simulink model "Improved_version_succesful1"  (Simulink 7.3)
settings: Solver=ode45  StartTime=0.0  StopTime=.25  RelTol=1e-3
undefined symbols (not defined in the file or in its folder): x
libraries: powerlib x176, powerlib_extras x116
(part 2 of 3)

== system Improved_version_succesful1/compensation section3/compensation block ==
  vL : Inport  OutDataType=fixdt(1, 16)  OutScaling=2^0
  PL : Inport  Port=2  OutDataType=fixdt(1, 16)  OutScaling=2^0
  iL : Inport  Port=3  OutDataType=fixdt(1, 16)  OutScaling=2^0
  1 constant power : Subsystem
  1st- : powerlib_extras/Control  Blocks/1st-Order  Filter  DialogController=POWERSYS.PowerSysDialog  SystemSampleTime=-1  FilterType=Lowpass  Tc=.00051  Initialize=off  Vac_Init=[0.8 -25 60]  Vdc_Init=-0.4  PlotResponse=off  param1=[1 500 1]
  1st-O : powerlib_extras/Control  Blocks/1st-Order  Filter  DialogController=POWERSYS.PowerSysDialog  SystemSampleTime=-1  FilterType=Lowpass  Tc=.00051  Initialize=off  Vac_Init=[0.8 -25 60]  Vdc_Init=-0.4  PlotResponse=off  param1=[1 500 1]
  1st-Order  Filter{,1,3,5..6} (5 alike) : powerlib_extras/Control  Blocks/1st-Order  Filter  DialogController=POWERSYS.PowerSysDialog  SystemSampleTime=-1  FilterType=Lowpass  Tc=.00051  Initialize=off  Vac_Init=[0.8 -25 60]  Vdc_Init=-0.4  PlotResponse=off  param1=[1 500 1]
  2 unity PF : Subsystem
  "3 balanced currents " : Subsystem
  Demux1 : Demux  Outputs=3
  Demux2 : Demux  Outputs=3
  Gain : Gain  Gain=x(6)*(1-x(5))  ParameterDataType=fixdt(1, 16)  ParameterScaling=2^0  OutDataType=fixdt(1, 16)  OutScaling=2^0
  Gain1 : Gain  Gain=x(5)*(1-x(6))  ParameterDataType=fixdt(1, 16)  ParameterScaling=2^0  OutDataType=fixdt(1, 16)  OutScaling=2^0
  Gain2 : Gain  Gain=x(5)*x(6)  ParameterDataType=fixdt(1, 16)  ParameterScaling=2^0  OutDataType=fixdt(1, 16)  OutScaling=2^0
  Mux1 : Mux  Inputs=3
  Mux2 : Mux  Inputs=3
  Mux3 : Mux  Inputs=3
  Saturation1 : Saturate  UpperLimit=100  LowerLimit=-100  OutDataType=sfix(16)  OutScaling=2^0
  Saturation2 : Saturate  UpperLimit=10000  LowerLimit=0  OutDataType=sfix(16)  OutScaling=2^0
  Saturation3 : Saturate  UpperLimit=500  LowerLimit=-500  OutDataType=sfix(16)  OutScaling=2^0
  Scope : Scope  NumInputPorts=3
      settings: YMin=-7.5~-1~-1  YMax=10~1~1  SaveName=ScopeData33
  Sum : Sum  Inputs=|+++  OutDataType=fixdt(1, 16)  OutScaling=2^0
  Icomp. : Outport  OutDataType=sfix(16)  OutScaling=2^0
  wires:
  vL/1 -> Saturation3/1
  Demux1/1 -> 1st-/1
  Demux1/2 -> 1st-Order  Filter3/1
  Demux1/3 -> 1st-Order  Filter/1
  Saturation1/1 -> Demux1/1
  1st-Order  Filter1/1 -> Mux3/3
  Demux2/1 -> 1st-O/1
  Demux2/2 -> 1st-Order  Filter5/1
  Demux2/3 -> 1st-Order  Filter1/1
  1st-O/1 -> Mux3/1
  1st-Order  Filter5/1 -> Mux3/2
  Saturation2/1 -> 1st-Order  Filter6/1
  1st-/1 -> Mux2/1
  1st-Order  Filter3/1 -> Mux2/2
  1st-Order  Filter/1 -> Mux2/3
  Saturation3/1 -> Demux2/1
  iL/1 -> Saturation1/1
  PL/1 -> Saturation2/1
  Mux3/1 -> Mux1/2
  Mux2/1 -> Mux1/1
  1st-Order  Filter6/1 -> Mux1/3
  Gain/1 -> 1 constant power/1(In1)
  Mux1/1 -> Gain/1, Gain1/1, Gain2/1
  Gain1/1 -> 2 unity PF/1(In1)
  1 constant power/1(Out2) -> Sum/1, Scope/1
  2 unity PF/1(Out1) -> Sum/2, Scope/2
  Gain2/1 -> "3 balanced currents "/1(In1)
  "3 balanced currents "/1(iCabc) -> Sum/3, Scope/3
  Sum/1 -> Icomp./1

== system Improved_version_succesful1/compensation section4/compensation block ==
  vL : Inport  OutDataType=fixdt(1, 16)  OutScaling=2^0
  PL : Inport  Port=2  OutDataType=fixdt(1, 16)  OutScaling=2^0
  iL : Inport  Port=3  OutDataType=fixdt(1, 16)  OutScaling=2^0
  1 constant power : Subsystem
  1st- : powerlib_extras/Control  Blocks/1st-Order  Filter  DialogController=POWERSYS.PowerSysDialog  SystemSampleTime=-1  FilterType=Lowpass  Tc=.00051  Initialize=off  Vac_Init=[0.8 -25 60]  Vdc_Init=-0.4  PlotResponse=off  param1=[1 500 1]
  1st-O : powerlib_extras/Control  Blocks/1st-Order  Filter  DialogController=POWERSYS.PowerSysDialog  SystemSampleTime=-1  FilterType=Lowpass  Tc=.00051  Initialize=off  Vac_Init=[0.8 -25 60]  Vdc_Init=-0.4  PlotResponse=off  param1=[1 500 1]
  1st-Order  Filter{,1,3,5..6} (5 alike) : powerlib_extras/Control  Blocks/1st-Order  Filter  DialogController=POWERSYS.PowerSysDialog  SystemSampleTime=-1  FilterType=Lowpass  Tc=.00051  Initialize=off  Vac_Init=[0.8 -25 60]  Vdc_Init=-0.4  PlotResponse=off  param1=[1 500 1]
  2 unity PF : Subsystem
  "3 balanced currents " : Subsystem
  Demux1 : Demux  Outputs=3
  Demux2 : Demux  Outputs=3
  Gain : Gain  Gain=x(8)*(1-x(7))  ParameterDataType=fixdt(1, 16)  ParameterScaling=2^0  OutDataType=fixdt(1, 16)  OutScaling=2^0
  Gain1 : Gain  Gain=x(7)*(1-x(8))  ParameterDataType=fixdt(1, 16)  ParameterScaling=2^0  OutDataType=fixdt(1, 16)  OutScaling=2^0
  Gain2 : Gain  Gain=x(7)*x(8)  ParameterDataType=fixdt(1, 16)  ParameterScaling=2^0  OutDataType=fixdt(1, 16)  OutScaling=2^0
  Mux1 : Mux  Inputs=3
  Mux2 : Mux  Inputs=3
  Mux3 : Mux  Inputs=3
  Saturation1 : Saturate  UpperLimit=100  LowerLimit=-100  OutDataType=sfix(16)  OutScaling=2^0
  Saturation2 : Saturate  UpperLimit=10000  LowerLimit=0  OutDataType=sfix(16)  OutScaling=2^0
  Saturation3 : Saturate  UpperLimit=500  LowerLimit=-500  OutDataType=sfix(16)  OutScaling=2^0
  Scope : Scope  NumInputPorts=3
      settings: YMin=-7.5~-1~-1  YMax=10~1~1  SaveName=ScopeData33
  Sum : Sum  Inputs=|+++  OutDataType=fixdt(1, 16)  OutScaling=2^0
  Icomp. : Outport  OutDataType=sfix(16)  OutScaling=2^0
  wires:
  Sum/1 -> Icomp./1
  "3 balanced currents "/1(iCabc) -> Scope/3, Sum/3
  Gain2/1 -> "3 balanced currents "/1(In1)
  2 unity PF/1(Out1) -> Scope/2, Sum/2
  1 constant power/1(Out2) -> Scope/1, Sum/1
  Gain1/1 -> 2 unity PF/1(In1)
  Mux1/1 -> Gain2/1, Gain1/1, Gain/1
  Gain/1 -> 1 constant power/1(In1)
  1st-Order  Filter6/1 -> Mux1/3
  Mux2/1 -> Mux1/1
  Mux3/1 -> Mux1/2
  PL/1 -> Saturation2/1
  iL/1 -> Saturation1/1
  Saturation3/1 -> Demux2/1
  1st-Order  Filter/1 -> Mux2/3
  1st-Order  Filter3/1 -> Mux2/2
  1st-/1 -> Mux2/1
  Saturation2/1 -> 1st-Order  Filter6/1
  1st-Order  Filter5/1 -> Mux3/2
  1st-O/1 -> Mux3/1
  Demux2/3 -> 1st-Order  Filter1/1
  Demux2/2 -> 1st-Order  Filter5/1
  Demux2/1 -> 1st-O/1
  1st-Order  Filter1/1 -> Mux3/3
  Saturation1/1 -> Demux1/1
  Demux1/3 -> 1st-Order  Filter/1
  Demux1/2 -> 1st-Order  Filter3/1
  Demux1/1 -> 1st-/1
  vL/1 -> Saturation3/1

== system Improved_version_succesful1/compensation section5/compensation block ==
  vL : Inport  OutDataType=fixdt(1, 16)  OutScaling=2^0
  PL : Inport  Port=2  OutDataType=fixdt(1, 16)  OutScaling=2^0
  iL : Inport  Port=3  OutDataType=fixdt(1, 16)  OutScaling=2^0
  1 constant power : Subsystem
  1st- : powerlib_extras/Control  Blocks/1st-Order  Filter  DialogController=POWERSYS.PowerSysDialog  SystemSampleTime=-1  FilterType=Lowpass  Tc=.00051  Initialize=off  Vac_Init=[0.8 -25 60]  Vdc_Init=-0.4  PlotResponse=off  param1=[1 500 1]
  1st-O : powerlib_extras/Control  Blocks/1st-Order  Filter  DialogController=POWERSYS.PowerSysDialog  SystemSampleTime=-1  FilterType=Lowpass  Tc=.00051  Initialize=off  Vac_Init=[0.8 -25 60]  Vdc_Init=-0.4  PlotResponse=off  param1=[1 500 1]
  1st-Order  Filter{,1,3,5..6} (5 alike) : powerlib_extras/Control  Blocks/1st-Order  Filter  DialogController=POWERSYS.PowerSysDialog  SystemSampleTime=-1  FilterType=Lowpass  Tc=.00051  Initialize=off  Vac_Init=[0.8 -25 60]  Vdc_Init=-0.4  PlotResponse=off  param1=[1 500 1]
  2 unity PF : Subsystem
  "3 balanced currents " : Subsystem
  Demux1 : Demux  Outputs=3
  Demux2 : Demux  Outputs=3
  Gain : Gain  Gain=x(10)*(1-x(9))  ParameterDataType=fixdt(1, 16)  ParameterScaling=2^0  OutDataType=fixdt(1, 16)  OutScaling=2^0
  Gain1 : Gain  Gain=x(9)*(1-x(10))  ParameterDataType=fixdt(1, 16)  ParameterScaling=2^0  OutDataType=fixdt(1, 16)  OutScaling=2^0
  Gain2 : Gain  Gain=x(9)*x(10)  ParameterDataType=fixdt(1, 16)  ParameterScaling=2^0  OutDataType=fixdt(1, 16)  OutScaling=2^0
  Mux1 : Mux  Inputs=3
  Mux2 : Mux  Inputs=3
  Mux3 : Mux  Inputs=3
  Saturation1 : Saturate  UpperLimit=100  LowerLimit=-100  OutDataType=sfix(16)  OutScaling=2^0
  Saturation2 : Saturate  UpperLimit=10000  LowerLimit=0  OutDataType=sfix(16)  OutScaling=2^0
  Saturation3 : Saturate  UpperLimit=500  LowerLimit=-500  OutDataType=sfix(16)  OutScaling=2^0
  Scope : Scope  NumInputPorts=3
      settings: YMin=-7.5~-1~-1  YMax=10~1~1  SaveName=ScopeData33
  Sum : Sum  Inputs=|+++  OutDataType=fixdt(1, 16)  OutScaling=2^0
  Icomp. : Outport  OutDataType=sfix(16)  OutScaling=2^0
  wires:
  vL/1 -> Saturation3/1
  Demux1/1 -> 1st-/1
  Demux1/2 -> 1st-Order  Filter3/1
  Demux1/3 -> 1st-Order  Filter/1
  Saturation1/1 -> Demux1/1
  1st-Order  Filter1/1 -> Mux3/3
  Demux2/1 -> 1st-O/1
  Demux2/2 -> 1st-Order  Filter5/1
  Demux2/3 -> 1st-Order  Filter1/1
  1st-O/1 -> Mux3/1
  1st-Order  Filter5/1 -> Mux3/2
  Saturation2/1 -> 1st-Order  Filter6/1
  1st-/1 -> Mux2/1
  1st-Order  Filter3/1 -> Mux2/2
  1st-Order  Filter/1 -> Mux2/3
  Saturation3/1 -> Demux2/1
  iL/1 -> Saturation1/1
  PL/1 -> Saturation2/1
  Mux3/1 -> Mux1/2
  Mux2/1 -> Mux1/1
  1st-Order  Filter6/1 -> Mux1/3
  Gain/1 -> 1 constant power/1(In1)
  Mux1/1 -> Gain/1, Gain1/1, Gain2/1
  Gain1/1 -> 2 unity PF/1(In1)
  1 constant power/1(Out2) -> Sum/1, Scope/1
  2 unity PF/1(Out1) -> Sum/2, Scope/2
  Gain2/1 -> "3 balanced currents "/1(In1)
  "3 balanced currents "/1(iCabc) -> Sum/3, Scope/3
  Sum/1 -> Icomp./1

== system Improved_version_succesful1/compensation section1/compensation block/1 constant power ==
  In1 : Inport  OutDataType=fixdt(1, 16)  OutScaling=2^0
  Demux : Demux  Outputs=3
  Demux1 : Demux  Outputs=7
  Discrete  Mean value : powerlib_extras/Discrete Measurements/Discrete  Mean value  DialogController=POWERSYS.PowerSysDialog  SystemSampleTime=-1  Freq=50  Vinit=.001  Ts=50e-6
  Embedded MATLAB Function : Stateflow chart  TreatAsAtomicUnit=on
  Embedded MATLAB Function1 : Stateflow chart  TreatAsAtomicUnit=on
  Embedded MATLAB Function3 : Stateflow chart  TreatAsAtomicUnit=on
  Embedded MATLAB Function4 : Stateflow chart  TreatAsAtomicUnit=on
  Mux1 : Mux  Inputs=3
  Mux3 : Mux  Inputs=3
  Mux4 : Mux  Inputs=3
  Scope1 : Scope  NumInputPorts=3
      settings: YMin=-1~-1~-1  YMax=1~1~1  SaveName=ScopeData32
  Out2 : Outport  OutDataType=sfix(16)  OutScaling=2^0
  wires:
  Mux3/1 -> Embedded MATLAB Function/1(a)
  Mux4/1 -> Embedded MATLAB Function1/1(b)
  Embedded MATLAB Function3/1(y) -> Demux/1, Out2/1
  Embedded MATLAB Function4/1(y) -> Embedded MATLAB Function3/1(h)
  Mux1/1 -> Embedded MATLAB Function4/1(a)
  Discrete  Mean value/1 -> Mux1/2
  Embedded MATLAB Function1/1(y) -> Mux1/1
  Demux/3 -> Scope1/3
  Demux/2 -> Scope1/2
  Demux/1 -> Scope1/1
  Embedded MATLAB Function/1(y) -> Mux1/3
  In1/1 -> Demux1/1
  Demux1/1 -> Mux3/1
  Demux1/2 -> Mux3/2
  Demux1/3 -> Mux3/3
  Demux1/4 -> Mux4/1
  Demux1/5 -> Mux4/2
  Demux1/6 -> Mux4/3
  Demux1/7 -> Discrete  Mean value/1

== system Improved_version_succesful1/compensation section1/compensation block/2 unity PF ==
  In1 : Inport  OutDataType=fixdt(1, 16)  OutScaling=2^0
  Demux : Demux  Outputs=3
  Demux1 : Demux  Outputs=7
  Discrete  Mean value : powerlib_extras/Discrete Measurements/Discrete  Mean value  DialogController=POWERSYS.PowerSysDialog  SystemSampleTime=-1  Freq=50  Vinit=0  Ts=50e-6
  Discrete  Mean value1 : powerlib_extras/Discrete Measurements/Discrete  Mean value  DialogController=POWERSYS.PowerSysDialog  SystemSampleTime=-1  Freq=50  Vinit=0  Ts=50e-6
  Embedded MATLAB Function : Stateflow chart  TreatAsAtomicUnit=on
  Embedded MATLAB Function1 : Stateflow chart  TreatAsAtomicUnit=on
  Embedded MATLAB Function2 : Stateflow chart  TreatAsAtomicUnit=on
  Embedded MATLAB Function3 : Stateflow chart  TreatAsAtomicUnit=on
  Embedded MATLAB Function4 : Stateflow chart  TreatAsAtomicUnit=on
  Mux1 : Mux
  Mux3 : Mux  Inputs=3
  Mux4 : Mux  Inputs=3
  Scope : Scope  NumInputPorts=3
      settings: YMin=-1~-1~-1  YMax=1~1~1  SaveName=ScopeData31
  Out1 : Outport  OutDataType=sfix(16)  OutScaling=2^0
  wires:
  Embedded MATLAB Function1/1(y) -> Embedded MATLAB Function2/1(a), Mux1/2
  Demux1/7 -> Discrete  Mean value/1
  Mux4/1 -> Embedded MATLAB Function1/1(b)
  Mux3/1 -> Embedded MATLAB Function/1(a)
  Demux1/6 -> Mux4/3
  Demux1/5 -> Mux4/2
  Demux1/4 -> Mux4/1
  Demux1/3 -> Mux3/3
  Demux1/2 -> Mux3/2
  Demux1/1 -> Mux3/1
  In1/1 -> Demux1/1
  Embedded MATLAB Function/1(y) -> Mux1/1
  Discrete  Mean value1/1 -> Mux1/3
  Embedded MATLAB Function2/1(y) -> Discrete  Mean value1/1
  Embedded MATLAB Function3/1(y) -> Out1/1, Demux/1
  Embedded MATLAB Function4/1(y) -> Embedded MATLAB Function3/1(h)
  Mux1/1 -> Embedded MATLAB Function4/1(a)
  Discrete  Mean value/1 -> Mux1/4
  Demux/3 -> Scope/3
  Demux/2 -> Scope/2
  Demux/1 -> Scope/1

== system Improved_version_succesful1/compensation section1/compensation block/3 balanced currents  ==
  In1 : Inport  OutDataType=fixdt(1, 16)  OutScaling=2^0
  Demux1 : Demux  Outputs=7
  Embedded MATLAB Function : Stateflow chart  TreatAsAtomicUnit=on
  Embedded MATLAB Function2 : Stateflow chart  TreatAsAtomicUnit=on
  Embedded MATLAB Function3 : Stateflow chart  TreatAsAtomicUnit=on
  Mean Value : powerlib_extras/Measurements/Mean Value  DialogController=POWERSYS.PowerSysDialog  SystemSampleTime=-1  Period=1/60
  Mux2 : Mux
  Mux3 : Mux  Inputs=3
  Mux4 : Mux  Inputs=3
  Saturation : Saturate  UpperLimit=100  LowerLimit=-100  OutDataType=sfix(16)  OutScaling=2^0
  Scope : Scope  NumInputPorts=2
      settings: YMin=-200~-1  YMax=200~1  SaveName=ScopeData34
  Scope1 : Scope  NumInputPorts=3
      settings: YMin=-30~-500~0  YMax=25~500~7000  SaveName=ScopeData35
  e0ab+1 : MATLABFcn  MATLABFcn=[1/sqrt(3) 1/sqrt(3) 1/sqrt(3); sqrt(2)/sqrt(3) -1/sqrt(6) -1/sqrt(6); 0 1/sqrt(2) -1/sqrt(2)]*u
  positive sequence1 : Subsystem
  iCabc : Outport  OutDataType=fixdt(1, 16)  OutScaling=2^0
  wires:
  In1/1 -> Demux1/1
  Demux1/1 -> Mux3/1
  Demux1/2 -> Mux3/2
  Demux1/3 -> Mux3/3
  Demux1/4 -> Mux4/1
  Demux1/5 -> Mux4/2
  Demux1/6 -> Mux4/3
  Embedded MATLAB Function/1(iL_0dq) -> Mux2/1
  e0ab+1/1 -> Mux2/2
  Mean Value/1 -> Mux2/4
  Mux2/1 -> Embedded MATLAB Function2/1(u)
  Embedded MATLAB Function2/1(iL_0dq) -> Embedded MATLAB Function3/1(u)
  Embedded MATLAB Function3/1(y) -> Saturation/1
  positive sequence1/2(E+^2) -> Mux2/3
  positive sequence1/1(eabc1+) -> e0ab+1/1
  Saturation/1 -> iCabc/1, Scope/1
  Mux3/1 -> Embedded MATLAB Function/1(u), Scope1/1
  Mux4/1 -> positive sequence1/1(In1), Scope1/2
  Demux1/7 -> Mean Value/1, Scope1/3

== system Improved_version_succesful1/compensation section2/compensation block/1 constant power ==
  In1 : Inport  OutDataType=fixdt(1, 16)  OutScaling=2^0
  Demux : Demux  Outputs=3
  Demux1 : Demux  Outputs=7
  Discrete  Mean value : powerlib_extras/Discrete Measurements/Discrete  Mean value  DialogController=POWERSYS.PowerSysDialog  SystemSampleTime=-1  Freq=50  Vinit=.001  Ts=50e-6
  Embedded MATLAB Function : Stateflow chart  TreatAsAtomicUnit=on
  Embedded MATLAB Function1 : Stateflow chart  TreatAsAtomicUnit=on
  Embedded MATLAB Function3 : Stateflow chart  TreatAsAtomicUnit=on
  Embedded MATLAB Function4 : Stateflow chart  TreatAsAtomicUnit=on
  Mux1 : Mux  Inputs=3
  Mux3 : Mux  Inputs=3
  Mux4 : Mux  Inputs=3
  Scope1 : Scope  NumInputPorts=3
      settings: YMin=-1~-1~-1  YMax=1~1~1  SaveName=ScopeData32
  Out2 : Outport  OutDataType=sfix(16)  OutScaling=2^0
  wires:
  Demux1/7 -> Discrete  Mean value/1
  Demux1/6 -> Mux4/3
  Demux1/5 -> Mux4/2
  Demux1/4 -> Mux4/1
  Demux1/3 -> Mux3/3
  Demux1/2 -> Mux3/2
  Demux1/1 -> Mux3/1
  In1/1 -> Demux1/1
  Embedded MATLAB Function/1(y) -> Mux1/3
  Demux/1 -> Scope1/1
  Demux/2 -> Scope1/2
  Demux/3 -> Scope1/3
  Embedded MATLAB Function1/1(y) -> Mux1/1
  Discrete  Mean value/1 -> Mux1/2
  Mux1/1 -> Embedded MATLAB Function4/1(a)
  Embedded MATLAB Function4/1(y) -> Embedded MATLAB Function3/1(h)
  Embedded MATLAB Function3/1(y) -> Out2/1, Demux/1
  Mux4/1 -> Embedded MATLAB Function1/1(b)
  Mux3/1 -> Embedded MATLAB Function/1(a)

== system Improved_version_succesful1/compensation section2/compensation block/2 unity PF ==
  In1 : Inport  OutDataType=fixdt(1, 16)  OutScaling=2^0
  Demux : Demux  Outputs=3
  Demux1 : Demux  Outputs=7
  Discrete  Mean value : powerlib_extras/Discrete Measurements/Discrete  Mean value  DialogController=POWERSYS.PowerSysDialog  SystemSampleTime=-1  Freq=50  Vinit=0  Ts=50e-6
  Discrete  Mean value1 : powerlib_extras/Discrete Measurements/Discrete  Mean value  DialogController=POWERSYS.PowerSysDialog  SystemSampleTime=-1  Freq=50  Vinit=0  Ts=50e-6
  Embedded MATLAB Function : Stateflow chart  TreatAsAtomicUnit=on
  Embedded MATLAB Function1 : Stateflow chart  TreatAsAtomicUnit=on
  Embedded MATLAB Function2 : Stateflow chart  TreatAsAtomicUnit=on
  Embedded MATLAB Function3 : Stateflow chart  TreatAsAtomicUnit=on
  Embedded MATLAB Function4 : Stateflow chart  TreatAsAtomicUnit=on
  Mux1 : Mux
  Mux3 : Mux  Inputs=3
  Mux4 : Mux  Inputs=3
  Scope : Scope  NumInputPorts=3
      settings: YMin=-1~-1~-1  YMax=1~1~1  SaveName=ScopeData31
  Out1 : Outport  OutDataType=sfix(16)  OutScaling=2^0
  wires:
  Demux/1 -> Scope/1
  Demux/2 -> Scope/2
  Demux/3 -> Scope/3
  Discrete  Mean value/1 -> Mux1/4
  Mux1/1 -> Embedded MATLAB Function4/1(a)
  Embedded MATLAB Function4/1(y) -> Embedded MATLAB Function3/1(h)
  Embedded MATLAB Function3/1(y) -> Demux/1, Out1/1
  Embedded MATLAB Function2/1(y) -> Discrete  Mean value1/1
  Discrete  Mean value1/1 -> Mux1/3
  Embedded MATLAB Function/1(y) -> Mux1/1
  In1/1 -> Demux1/1
  Demux1/1 -> Mux3/1
  Demux1/2 -> Mux3/2
  Demux1/3 -> Mux3/3
  Demux1/4 -> Mux4/1
  Demux1/5 -> Mux4/2
  Demux1/6 -> Mux4/3
  Mux3/1 -> Embedded MATLAB Function/1(a)
  Mux4/1 -> Embedded MATLAB Function1/1(b)
  Demux1/7 -> Discrete  Mean value/1
  Embedded MATLAB Function1/1(y) -> Mux1/2, Embedded MATLAB Function2/1(a)

== system Improved_version_succesful1/compensation section2/compensation block/3 balanced currents  ==
  In1 : Inport  OutDataType=fixdt(1, 16)  OutScaling=2^0
  Demux1 : Demux  Outputs=7
  Embedded MATLAB Function : Stateflow chart  TreatAsAtomicUnit=on
  Embedded MATLAB Function2 : Stateflow chart  TreatAsAtomicUnit=on
  Embedded MATLAB Function3 : Stateflow chart  TreatAsAtomicUnit=on
  Mean Value : powerlib_extras/Measurements/Mean Value  DialogController=POWERSYS.PowerSysDialog  SystemSampleTime=-1  Period=1/60
  Mux2 : Mux
  Mux3 : Mux  Inputs=3
  Mux4 : Mux  Inputs=3
  Saturation : Saturate  UpperLimit=100  LowerLimit=-100  OutDataType=sfix(16)  OutScaling=2^0
  Scope : Scope  NumInputPorts=2
      settings: YMin=-200~-1  YMax=200~1  SaveName=ScopeData34
  Scope1 : Scope  NumInputPorts=3
      settings: YMin=-30~-500~0  YMax=25~500~7000  SaveName=ScopeData35
  e0ab+1 : MATLABFcn  MATLABFcn=[1/sqrt(3) 1/sqrt(3) 1/sqrt(3); sqrt(2)/sqrt(3) -1/sqrt(6) -1/sqrt(6); 0 1/sqrt(2) -1/sqrt(2)]*u
  positive sequence1 : Subsystem
  iCabc : Outport  OutDataType=fixdt(1, 16)  OutScaling=2^0
  wires:
  Demux1/7 -> Scope1/3, Mean Value/1
  Mux4/1 -> Scope1/2, positive sequence1/1(In1)
  Mux3/1 -> Scope1/1, Embedded MATLAB Function/1(u)
  Saturation/1 -> Scope/1, iCabc/1
  positive sequence1/1(eabc1+) -> e0ab+1/1
  positive sequence1/2(E+^2) -> Mux2/3
  Embedded MATLAB Function3/1(y) -> Saturation/1
  Embedded MATLAB Function2/1(iL_0dq) -> Embedded MATLAB Function3/1(u)
  Mux2/1 -> Embedded MATLAB Function2/1(u)
  Mean Value/1 -> Mux2/4
  e0ab+1/1 -> Mux2/2
  Embedded MATLAB Function/1(iL_0dq) -> Mux2/1
  Demux1/6 -> Mux4/3
  Demux1/5 -> Mux4/2
  Demux1/4 -> Mux4/1
  Demux1/3 -> Mux3/3
  Demux1/2 -> Mux3/2
  Demux1/1 -> Mux3/1
  In1/1 -> Demux1/1

== system Improved_version_succesful1/compensation section3/compensation block/1 constant power ==
  In1 : Inport  OutDataType=fixdt(1, 16)  OutScaling=2^0
  Demux : Demux  Outputs=3
  Demux1 : Demux  Outputs=7
  Discrete  Mean value : powerlib_extras/Discrete Measurements/Discrete  Mean value  DialogController=POWERSYS.PowerSysDialog  SystemSampleTime=-1  Freq=50  Vinit=.001  Ts=50e-6
  Embedded MATLAB Function : Stateflow chart  TreatAsAtomicUnit=on
  Embedded MATLAB Function1 : Stateflow chart  TreatAsAtomicUnit=on
  Embedded MATLAB Function3 : Stateflow chart  TreatAsAtomicUnit=on
  Embedded MATLAB Function4 : Stateflow chart  TreatAsAtomicUnit=on
  Mux1 : Mux  Inputs=3
  Mux3 : Mux  Inputs=3
  Mux4 : Mux  Inputs=3
  Scope1 : Scope  NumInputPorts=3
      settings: YMin=-1~-1~-1  YMax=1~1~1  SaveName=ScopeData32
  Out2 : Outport  OutDataType=sfix(16)  OutScaling=2^0
  wires:
  Mux3/1 -> Embedded MATLAB Function/1(a)
  Mux4/1 -> Embedded MATLAB Function1/1(b)
  Embedded MATLAB Function3/1(y) -> Demux/1, Out2/1
  Embedded MATLAB Function4/1(y) -> Embedded MATLAB Function3/1(h)
  Mux1/1 -> Embedded MATLAB Function4/1(a)
  Discrete  Mean value/1 -> Mux1/2
  Embedded MATLAB Function1/1(y) -> Mux1/1
  Demux/3 -> Scope1/3
  Demux/2 -> Scope1/2
  Demux/1 -> Scope1/1
  Embedded MATLAB Function/1(y) -> Mux1/3
  In1/1 -> Demux1/1
  Demux1/1 -> Mux3/1
  Demux1/2 -> Mux3/2
  Demux1/3 -> Mux3/3
  Demux1/4 -> Mux4/1
  Demux1/5 -> Mux4/2
  Demux1/6 -> Mux4/3
  Demux1/7 -> Discrete  Mean value/1

== system Improved_version_succesful1/compensation section3/compensation block/2 unity PF ==
  In1 : Inport  OutDataType=fixdt(1, 16)  OutScaling=2^0
  Demux : Demux  Outputs=3
  Demux1 : Demux  Outputs=7
  Discrete  Mean value : powerlib_extras/Discrete Measurements/Discrete  Mean value  DialogController=POWERSYS.PowerSysDialog  SystemSampleTime=-1  Freq=50  Vinit=0  Ts=50e-6
  Discrete  Mean value1 : powerlib_extras/Discrete Measurements/Discrete  Mean value  DialogController=POWERSYS.PowerSysDialog  SystemSampleTime=-1  Freq=50  Vinit=0  Ts=50e-6
  Embedded MATLAB Function : Stateflow chart  TreatAsAtomicUnit=on
  Embedded MATLAB Function1 : Stateflow chart  TreatAsAtomicUnit=on
  Embedded MATLAB Function2 : Stateflow chart  TreatAsAtomicUnit=on
  Embedded MATLAB Function3 : Stateflow chart  TreatAsAtomicUnit=on
  Embedded MATLAB Function4 : Stateflow chart  TreatAsAtomicUnit=on
  Mux1 : Mux
  Mux3 : Mux  Inputs=3
  Mux4 : Mux  Inputs=3
  Scope : Scope  NumInputPorts=3
      settings: YMin=-1~-1~-1  YMax=1~1~1  SaveName=ScopeData31
  Out1 : Outport  OutDataType=sfix(16)  OutScaling=2^0
  wires:
  Embedded MATLAB Function1/1(y) -> Embedded MATLAB Function2/1(a), Mux1/2
  Demux1/7 -> Discrete  Mean value/1
  Mux4/1 -> Embedded MATLAB Function1/1(b)
  Mux3/1 -> Embedded MATLAB Function/1(a)
  Demux1/6 -> Mux4/3
  Demux1/5 -> Mux4/2
  Demux1/4 -> Mux4/1
  Demux1/3 -> Mux3/3
  Demux1/2 -> Mux3/2
  Demux1/1 -> Mux3/1
  In1/1 -> Demux1/1
  Embedded MATLAB Function/1(y) -> Mux1/1
  Discrete  Mean value1/1 -> Mux1/3
  Embedded MATLAB Function2/1(y) -> Discrete  Mean value1/1
  Embedded MATLAB Function3/1(y) -> Out1/1, Demux/1
  Embedded MATLAB Function4/1(y) -> Embedded MATLAB Function3/1(h)
  Mux1/1 -> Embedded MATLAB Function4/1(a)
  Discrete  Mean value/1 -> Mux1/4
  Demux/3 -> Scope/3
  Demux/2 -> Scope/2
  Demux/1 -> Scope/1

== system Improved_version_succesful1/compensation section3/compensation block/3 balanced currents  ==
  In1 : Inport  OutDataType=fixdt(1, 16)  OutScaling=2^0
  Demux1 : Demux  Outputs=7
  Embedded MATLAB Function : Stateflow chart  TreatAsAtomicUnit=on
  Embedded MATLAB Function2 : Stateflow chart  TreatAsAtomicUnit=on
  Embedded MATLAB Function3 : Stateflow chart  TreatAsAtomicUnit=on
  Mean Value : powerlib_extras/Measurements/Mean Value  DialogController=POWERSYS.PowerSysDialog  SystemSampleTime=-1  Period=1/60
  Mux2 : Mux
  Mux3 : Mux  Inputs=3
  Mux4 : Mux  Inputs=3
  Saturation : Saturate  UpperLimit=100  LowerLimit=-100  OutDataType=sfix(16)  OutScaling=2^0
  Scope : Scope  NumInputPorts=2
      settings: YMin=-200~-1  YMax=200~1  SaveName=ScopeData34
  Scope1 : Scope  NumInputPorts=3
      settings: YMin=-30~-500~0  YMax=25~500~7000  SaveName=ScopeData35
  e0ab+1 : MATLABFcn  MATLABFcn=[1/sqrt(3) 1/sqrt(3) 1/sqrt(3); sqrt(2)/sqrt(3) -1/sqrt(6) -1/sqrt(6); 0 1/sqrt(2) -1/sqrt(2)]*u
  positive sequence1 : Subsystem
  iCabc : Outport  OutDataType=fixdt(1, 16)  OutScaling=2^0
  wires:
  In1/1 -> Demux1/1
  Demux1/1 -> Mux3/1
  Demux1/2 -> Mux3/2
  Demux1/3 -> Mux3/3
  Demux1/4 -> Mux4/1
  Demux1/5 -> Mux4/2
  Demux1/6 -> Mux4/3
  Embedded MATLAB Function/1(iL_0dq) -> Mux2/1
  e0ab+1/1 -> Mux2/2
  Mean Value/1 -> Mux2/4
  Mux2/1 -> Embedded MATLAB Function2/1(u)
  Embedded MATLAB Function2/1(iL_0dq) -> Embedded MATLAB Function3/1(u)
  Embedded MATLAB Function3/1(y) -> Saturation/1
  positive sequence1/2(E+^2) -> Mux2/3
  positive sequence1/1(eabc1+) -> e0ab+1/1
  Saturation/1 -> iCabc/1, Scope/1
  Mux3/1 -> Embedded MATLAB Function/1(u), Scope1/1
  Mux4/1 -> positive sequence1/1(In1), Scope1/2
  Demux1/7 -> Mean Value/1, Scope1/3

== system Improved_version_succesful1/compensation section4/compensation block/1 constant power ==
  In1 : Inport  OutDataType=fixdt(1, 16)  OutScaling=2^0
  Demux : Demux  Outputs=3
  Demux1 : Demux  Outputs=7
  Discrete  Mean value : powerlib_extras/Discrete Measurements/Discrete  Mean value  DialogController=POWERSYS.PowerSysDialog  SystemSampleTime=-1  Freq=50  Vinit=.001  Ts=50e-6
  Embedded MATLAB Function : Stateflow chart  TreatAsAtomicUnit=on
  Embedded MATLAB Function1 : Stateflow chart  TreatAsAtomicUnit=on
  Embedded MATLAB Function3 : Stateflow chart  TreatAsAtomicUnit=on
  Embedded MATLAB Function4 : Stateflow chart  TreatAsAtomicUnit=on
  Mux1 : Mux  Inputs=3
  Mux3 : Mux  Inputs=3
  Mux4 : Mux  Inputs=3
  Scope1 : Scope  NumInputPorts=3
      settings: YMin=-1~-1~-1  YMax=1~1~1  SaveName=ScopeData32
  Out2 : Outport  OutDataType=sfix(16)  OutScaling=2^0
  wires:
  Demux1/7 -> Discrete  Mean value/1
  Demux1/6 -> Mux4/3
  Demux1/5 -> Mux4/2
  Demux1/4 -> Mux4/1
  Demux1/3 -> Mux3/3
  Demux1/2 -> Mux3/2
  Demux1/1 -> Mux3/1
  In1/1 -> Demux1/1
  Embedded MATLAB Function/1(y) -> Mux1/3
  Demux/1 -> Scope1/1
  Demux/2 -> Scope1/2
  Demux/3 -> Scope1/3
  Embedded MATLAB Function1/1(y) -> Mux1/1
  Discrete  Mean value/1 -> Mux1/2
  Mux1/1 -> Embedded MATLAB Function4/1(a)
  Embedded MATLAB Function4/1(y) -> Embedded MATLAB Function3/1(h)
  Embedded MATLAB Function3/1(y) -> Out2/1, Demux/1
  Mux4/1 -> Embedded MATLAB Function1/1(b)
  Mux3/1 -> Embedded MATLAB Function/1(a)

== system Improved_version_succesful1/compensation section4/compensation block/2 unity PF ==
  In1 : Inport  OutDataType=fixdt(1, 16)  OutScaling=2^0
  Demux : Demux  Outputs=3
  Demux1 : Demux  Outputs=7
  Discrete  Mean value : powerlib_extras/Discrete Measurements/Discrete  Mean value  DialogController=POWERSYS.PowerSysDialog  SystemSampleTime=-1  Freq=50  Vinit=0  Ts=50e-6
  Discrete  Mean value1 : powerlib_extras/Discrete Measurements/Discrete  Mean value  DialogController=POWERSYS.PowerSysDialog  SystemSampleTime=-1  Freq=50  Vinit=0  Ts=50e-6
  Embedded MATLAB Function : Stateflow chart  TreatAsAtomicUnit=on
  Embedded MATLAB Function1 : Stateflow chart  TreatAsAtomicUnit=on
  Embedded MATLAB Function2 : Stateflow chart  TreatAsAtomicUnit=on
  Embedded MATLAB Function3 : Stateflow chart  TreatAsAtomicUnit=on
  Embedded MATLAB Function4 : Stateflow chart  TreatAsAtomicUnit=on
  Mux1 : Mux
  Mux3 : Mux  Inputs=3
  Mux4 : Mux  Inputs=3
  Scope : Scope  NumInputPorts=3
      settings: YMin=-1~-1~-1  YMax=1~1~1  SaveName=ScopeData31
  Out1 : Outport  OutDataType=sfix(16)  OutScaling=2^0
  wires:
  Demux/1 -> Scope/1
  Demux/2 -> Scope/2
  Demux/3 -> Scope/3
  Discrete  Mean value/1 -> Mux1/4
  Mux1/1 -> Embedded MATLAB Function4/1(a)
  Embedded MATLAB Function4/1(y) -> Embedded MATLAB Function3/1(h)
  Embedded MATLAB Function3/1(y) -> Demux/1, Out1/1
  Embedded MATLAB Function2/1(y) -> Discrete  Mean value1/1
  Discrete  Mean value1/1 -> Mux1/3
  Embedded MATLAB Function/1(y) -> Mux1/1
  In1/1 -> Demux1/1
  Demux1/1 -> Mux3/1
  Demux1/2 -> Mux3/2
  Demux1/3 -> Mux3/3
  Demux1/4 -> Mux4/1
  Demux1/5 -> Mux4/2
  Demux1/6 -> Mux4/3
  Mux3/1 -> Embedded MATLAB Function/1(a)
  Mux4/1 -> Embedded MATLAB Function1/1(b)
  Demux1/7 -> Discrete  Mean value/1
  Embedded MATLAB Function1/1(y) -> Mux1/2, Embedded MATLAB Function2/1(a)

== system Improved_version_succesful1/compensation section4/compensation block/3 balanced currents  ==
  In1 : Inport  OutDataType=fixdt(1, 16)  OutScaling=2^0
  Demux1 : Demux  Outputs=7
  Embedded MATLAB Function : Stateflow chart  TreatAsAtomicUnit=on
  Embedded MATLAB Function2 : Stateflow chart  TreatAsAtomicUnit=on
  Embedded MATLAB Function3 : Stateflow chart  TreatAsAtomicUnit=on
  Mean Value : powerlib_extras/Measurements/Mean Value  DialogController=POWERSYS.PowerSysDialog  SystemSampleTime=-1  Period=1/60
  Mux2 : Mux
  Mux3 : Mux  Inputs=3
  Mux4 : Mux  Inputs=3
  Saturation : Saturate  UpperLimit=100  LowerLimit=-100  OutDataType=sfix(16)  OutScaling=2^0
  Scope : Scope  NumInputPorts=2
      settings: YMin=-200~-1  YMax=200~1  SaveName=ScopeData34
  Scope1 : Scope  NumInputPorts=3
      settings: YMin=-30~-500~0  YMax=25~500~7000  SaveName=ScopeData35
  e0ab+1 : MATLABFcn  MATLABFcn=[1/sqrt(3) 1/sqrt(3) 1/sqrt(3); sqrt(2)/sqrt(3) -1/sqrt(6) -1/sqrt(6); 0 1/sqrt(2) -1/sqrt(2)]*u
  positive sequence1 : Subsystem
  iCabc : Outport  OutDataType=fixdt(1, 16)  OutScaling=2^0
  wires:
  Demux1/7 -> Scope1/3, Mean Value/1
  Mux4/1 -> Scope1/2, positive sequence1/1(In1)
  Mux3/1 -> Scope1/1, Embedded MATLAB Function/1(u)
  Saturation/1 -> Scope/1, iCabc/1
  positive sequence1/1(eabc1+) -> e0ab+1/1
  positive sequence1/2(E+^2) -> Mux2/3
  Embedded MATLAB Function3/1(y) -> Saturation/1
  Embedded MATLAB Function2/1(iL_0dq) -> Embedded MATLAB Function3/1(u)
  Mux2/1 -> Embedded MATLAB Function2/1(u)
  Mean Value/1 -> Mux2/4
  e0ab+1/1 -> Mux2/2
  Embedded MATLAB Function/1(iL_0dq) -> Mux2/1
  Demux1/6 -> Mux4/3
  Demux1/5 -> Mux4/2
  Demux1/4 -> Mux4/1
  Demux1/3 -> Mux3/3
  Demux1/2 -> Mux3/2
  Demux1/1 -> Mux3/1
  In1/1 -> Demux1/1

== system Improved_version_succesful1/compensation section5/compensation block/1 constant power ==
  In1 : Inport  OutDataType=fixdt(1, 16)  OutScaling=2^0
  Demux : Demux  Outputs=3
  Demux1 : Demux  Outputs=7
  Discrete  Mean value : powerlib_extras/Discrete Measurements/Discrete  Mean value  DialogController=POWERSYS.PowerSysDialog  SystemSampleTime=-1  Freq=50  Vinit=.001  Ts=50e-6
  Embedded MATLAB Function : Stateflow chart  TreatAsAtomicUnit=on
  Embedded MATLAB Function1 : Stateflow chart  TreatAsAtomicUnit=on
  Embedded MATLAB Function3 : Stateflow chart  TreatAsAtomicUnit=on
  Embedded MATLAB Function4 : Stateflow chart  TreatAsAtomicUnit=on
  Mux1 : Mux  Inputs=3
  Mux3 : Mux  Inputs=3
  Mux4 : Mux  Inputs=3
  Scope1 : Scope  NumInputPorts=3
      settings: YMin=-1~-1~-1  YMax=1~1~1  SaveName=ScopeData32
  Out2 : Outport  OutDataType=sfix(16)  OutScaling=2^0
  wires:
  Mux3/1 -> Embedded MATLAB Function/1(a)
  Mux4/1 -> Embedded MATLAB Function1/1(b)
  Embedded MATLAB Function3/1(y) -> Demux/1, Out2/1
  Embedded MATLAB Function4/1(y) -> Embedded MATLAB Function3/1(h)
  Mux1/1 -> Embedded MATLAB Function4/1(a)
  Discrete  Mean value/1 -> Mux1/2
  Embedded MATLAB Function1/1(y) -> Mux1/1
  Demux/3 -> Scope1/3
  Demux/2 -> Scope1/2
  Demux/1 -> Scope1/1
  Embedded MATLAB Function/1(y) -> Mux1/3
  In1/1 -> Demux1/1
  Demux1/1 -> Mux3/1
  Demux1/2 -> Mux3/2
  Demux1/3 -> Mux3/3
  Demux1/4 -> Mux4/1
  Demux1/5 -> Mux4/2
  Demux1/6 -> Mux4/3
  Demux1/7 -> Discrete  Mean value/1

== system Improved_version_succesful1/compensation section5/compensation block/2 unity PF ==
  In1 : Inport  OutDataType=fixdt(1, 16)  OutScaling=2^0
  Demux : Demux  Outputs=3
  Demux1 : Demux  Outputs=7
  Discrete  Mean value : powerlib_extras/Discrete Measurements/Discrete  Mean value  DialogController=POWERSYS.PowerSysDialog  SystemSampleTime=-1  Freq=50  Vinit=0  Ts=50e-6
  Discrete  Mean value1 : powerlib_extras/Discrete Measurements/Discrete  Mean value  DialogController=POWERSYS.PowerSysDialog  SystemSampleTime=-1  Freq=50  Vinit=0  Ts=50e-6
  Embedded MATLAB Function : Stateflow chart  TreatAsAtomicUnit=on
  Embedded MATLAB Function1 : Stateflow chart  TreatAsAtomicUnit=on
  Embedded MATLAB Function2 : Stateflow chart  TreatAsAtomicUnit=on
  Embedded MATLAB Function3 : Stateflow chart  TreatAsAtomicUnit=on
  Embedded MATLAB Function4 : Stateflow chart  TreatAsAtomicUnit=on
  Mux1 : Mux
  Mux3 : Mux  Inputs=3
  Mux4 : Mux  Inputs=3
  Scope : Scope  NumInputPorts=3
      settings: YMin=-1~-1~-1  YMax=1~1~1  SaveName=ScopeData31
  Out1 : Outport  OutDataType=sfix(16)  OutScaling=2^0
  wires:
  Embedded MATLAB Function1/1(y) -> Embedded MATLAB Function2/1(a), Mux1/2
  Demux1/7 -> Discrete  Mean value/1
  Mux4/1 -> Embedded MATLAB Function1/1(b)
  Mux3/1 -> Embedded MATLAB Function/1(a)
  Demux1/6 -> Mux4/3
  Demux1/5 -> Mux4/2
  Demux1/4 -> Mux4/1
  Demux1/3 -> Mux3/3
  Demux1/2 -> Mux3/2
  Demux1/1 -> Mux3/1
  In1/1 -> Demux1/1
  Embedded MATLAB Function/1(y) -> Mux1/1
  Discrete  Mean value1/1 -> Mux1/3
  Embedded MATLAB Function2/1(y) -> Discrete  Mean value1/1
  Embedded MATLAB Function3/1(y) -> Out1/1, Demux/1
  Embedded MATLAB Function4/1(y) -> Embedded MATLAB Function3/1(h)
  Mux1/1 -> Embedded MATLAB Function4/1(a)
  Discrete  Mean value/1 -> Mux1/4
  Demux/3 -> Scope/3
  Demux/2 -> Scope/2
  Demux/1 -> Scope/1

== system Improved_version_succesful1/compensation section5/compensation block/3 balanced currents  ==
  In1 : Inport  OutDataType=fixdt(1, 16)  OutScaling=2^0
  Demux1 : Demux  Outputs=7
  Embedded MATLAB Function : Stateflow chart  TreatAsAtomicUnit=on
  Embedded MATLAB Function2 : Stateflow chart  TreatAsAtomicUnit=on
  Embedded MATLAB Function3 : Stateflow chart  TreatAsAtomicUnit=on
  Mean Value : powerlib_extras/Measurements/Mean Value  DialogController=POWERSYS.PowerSysDialog  SystemSampleTime=-1  Period=1/60
  Mux2 : Mux
  Mux3 : Mux  Inputs=3
  Mux4 : Mux  Inputs=3
  Saturation : Saturate  UpperLimit=100  LowerLimit=-100  OutDataType=sfix(16)  OutScaling=2^0
  Scope : Scope  NumInputPorts=2
      settings: YMin=-200~-1  YMax=200~1  SaveName=ScopeData34
  Scope1 : Scope  NumInputPorts=3
      settings: YMin=-30~-500~0  YMax=25~500~7000  SaveName=ScopeData35
  e0ab+1 : MATLABFcn  MATLABFcn=[1/sqrt(3) 1/sqrt(3) 1/sqrt(3); sqrt(2)/sqrt(3) -1/sqrt(6) -1/sqrt(6); 0 1/sqrt(2) -1/sqrt(2)]*u
  positive sequence1 : Subsystem
  iCabc : Outport  OutDataType=fixdt(1, 16)  OutScaling=2^0
  wires:
  In1/1 -> Demux1/1
  Demux1/1 -> Mux3/1
  Demux1/2 -> Mux3/2
  Demux1/3 -> Mux3/3
  Demux1/4 -> Mux4/1
  Demux1/5 -> Mux4/2
  Demux1/6 -> Mux4/3
  Embedded MATLAB Function/1(iL_0dq) -> Mux2/1
  e0ab+1/1 -> Mux2/2
  Mean Value/1 -> Mux2/4
  Mux2/1 -> Embedded MATLAB Function2/1(u)
  Embedded MATLAB Function2/1(iL_0dq) -> Embedded MATLAB Function3/1(u)
  Embedded MATLAB Function3/1(y) -> Saturation/1
  positive sequence1/2(E+^2) -> Mux2/3
  positive sequence1/1(eabc1+) -> e0ab+1/1
  Saturation/1 -> iCabc/1, Scope/1
  Mux3/1 -> Embedded MATLAB Function/1(u), Scope1/1
  Mux4/1 -> positive sequence1/1(In1), Scope1/2
  Demux1/7 -> Mean Value/1, Scope1/3

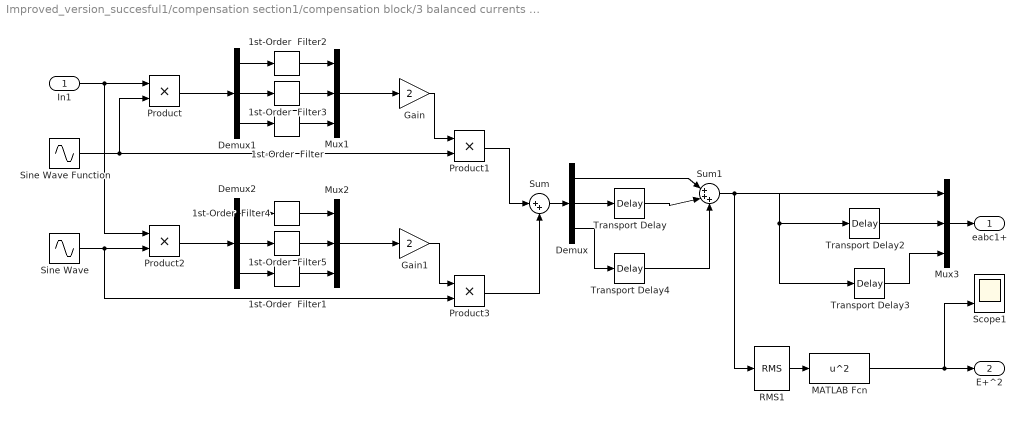
== system Improved_version_succesful1/compensation section1/compensation block/3 balanced currents /positive sequence1 ==
  In1 : Inport  OutDataType=sfix(16)  OutScaling=2^0
  1st-Order  Filter{,1,3,5} (4 alike) : powerlib_extras/Control  Blocks/1st-Order  Filter  DialogController=POWERSYS.PowerSysDialog  SystemSampleTime=-1  FilterType=Lowpass  Tc=.01  Initialize=off  Vac_Init=[0.8 -25 60]  Vdc_Init=-0.4  PlotResponse=off  param1=[1 500 1]
  1st-Order  Filter2 : powerlib_extras/Control  Blocks/1st-Order  Filter  DialogController=POWERSYS.PowerSysDialog  SystemSampleTime=-1  FilterType=Lowpass  Tc=.015  Initialize=off  Vac_Init=[0.8 -25 60]  Vdc_Init=-0.4  PlotResponse=off  param1=[1 500 1]
  1st-Order  Filter4 : powerlib_extras/Control  Blocks/1st-Order  Filter  DialogController=POWERSYS.PowerSysDialog  SystemSampleTime=-1  FilterType=Lowpass  Tc=.015  Initialize=off  Vac_Init=[0.8 -25 60]  Vdc_Init=-0.4  PlotResponse=off  param1=[1 500 1]
  Demux : Demux  Outputs=3
  Demux1 : Demux  Outputs=3
  Demux2 : Demux  Outputs=3
  Gain : Gain  Gain=2  ParameterDataType=sfix(16)  ParameterScaling=2^0  OutDataType=sfix(16)  OutScaling=2^0
  Gain1 : Gain  Gain=2  ParameterDataType=sfix(16)  ParameterScaling=2^0  OutDataType=sfix(16)  OutScaling=2^0
  MATLAB Fcn : MATLABFcn  MATLABFcn=u^2
  Mux1 : Mux  Inputs=3
  Mux2 : Mux  Inputs=3
  Mux3 : Mux  Inputs=3
  Product{,1..3} (4 alike) : Product  OutDataType=sfix(16)  OutScaling=2^0  RndMeth=Zero
  RMS1 : powerlib_extras/Measurements/RMS  DialogController=POWERSYS.PowerSysDialog  SystemSampleTime=-1  f1=50
  Scope1 : Scope  NumInputPorts=3
      settings: YMin=-1~-1~150000  YMax=1~1~320000
  Sine Wave : Sin  Amplitude=1  Bias=0  Frequency=100*pi  Phase=pi/2  Samples=10  SampleTime=0  Offset=0
  Sine Wave Function : Sin  Amplitude=1  Bias=0  Frequency=100*pi  Phase=0  Samples=10  SampleTime=0  Offset=0
  Sum : Sum  Inputs=|++  OutDataType=sfix(16)  OutScaling=2^0
  Sum1 : Sum  Inputs=|+++  OutDataType=sfix(16)  OutScaling=2^0
  Transport Delay : TransportDelay  DelayTime=.04/3
  Transport Delay2 : TransportDelay  DelayTime=.02/3
  Transport Delay3 : TransportDelay  DelayTime=.04/3
  Transport Delay4 : TransportDelay  DelayTime=.02/3
  eabc1+ : Outport  OutDataType=sfix(16)  OutScaling=2^0
  E+^2 : Outport  Port=2  OutDataType=sfix(16)  OutScaling=2^0
  wires:
  RMS1/1 -> MATLAB Fcn/1
  MATLAB Fcn/1 -> E+^2/1, Scope1/3
  In1/1 -> Product/1, Product2/1
  Sine Wave Function/1 -> Product/2, Product1/2
  1st-Order  Filter/1 -> Mux1/3
  Gain/1 -> Product1/1
  Sine Wave/1 -> Product2/2, Product3/2
  Gain1/1 -> Product3/1
  Product1/1 -> Sum/1
  Product3/1 -> Sum/2
  Sum/1 -> Demux/1
  Demux/2 -> Transport Delay/1
  Sum1/1 -> Transport Delay3/1, Mux3/1, RMS1/1, Transport Delay2/1
  Demux/3 -> Transport Delay4/1
  Transport Delay2/1 -> Mux3/2
  Transport Delay3/1 -> Mux3/3
  Mux3/1 -> eabc1+/1
  Demux1/1 -> 1st-Order  Filter2/1
  Demux1/2 -> 1st-Order  Filter3/1
  Demux1/3 -> 1st-Order  Filter/1
  Product/1 -> Demux1/1
  1st-Order  Filter2/1 -> Mux1/1
  1st-Order  Filter3/1 -> Mux1/2
  Mux1/1 -> Gain/1
  1st-Order  Filter1/1 -> Mux2/3
  Demux2/1 -> 1st-Order  Filter4/1
  Demux2/2 -> 1st-Order  Filter5/1
  Demux2/3 -> 1st-Order  Filter1/1
  Product2/1 -> Demux2/1
  1st-Order  Filter4/1 -> Mux2/1
  1st-Order  Filter5/1 -> Mux2/2
  Mux2/1 -> Gain1/1
  Demux/1 -> Sum1/1
  Transport Delay/1 -> Sum1/2
  Transport Delay4/1 -> Sum1/3

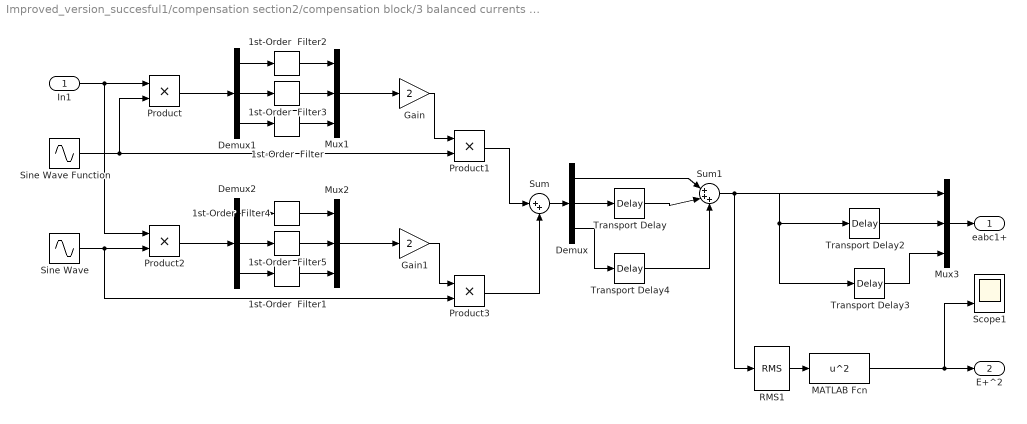
== system Improved_version_succesful1/compensation section2/compensation block/3 balanced currents /positive sequence1 ==
  In1 : Inport  OutDataType=sfix(16)  OutScaling=2^0
  1st-Order  Filter{,1,3,5} (4 alike) : powerlib_extras/Control  Blocks/1st-Order  Filter  DialogController=POWERSYS.PowerSysDialog  SystemSampleTime=-1  FilterType=Lowpass  Tc=.01  Initialize=off  Vac_Init=[0.8 -25 60]  Vdc_Init=-0.4  PlotResponse=off  param1=[1 500 1]
  1st-Order  Filter2 : powerlib_extras/Control  Blocks/1st-Order  Filter  DialogController=POWERSYS.PowerSysDialog  SystemSampleTime=-1  FilterType=Lowpass  Tc=.015  Initialize=off  Vac_Init=[0.8 -25 60]  Vdc_Init=-0.4  PlotResponse=off  param1=[1 500 1]
  1st-Order  Filter4 : powerlib_extras/Control  Blocks/1st-Order  Filter  DialogController=POWERSYS.PowerSysDialog  SystemSampleTime=-1  FilterType=Lowpass  Tc=.015  Initialize=off  Vac_Init=[0.8 -25 60]  Vdc_Init=-0.4  PlotResponse=off  param1=[1 500 1]
  Demux : Demux  Outputs=3
  Demux1 : Demux  Outputs=3
  Demux2 : Demux  Outputs=3
  Gain : Gain  Gain=2  ParameterDataType=sfix(16)  ParameterScaling=2^0  OutDataType=sfix(16)  OutScaling=2^0
  Gain1 : Gain  Gain=2  ParameterDataType=sfix(16)  ParameterScaling=2^0  OutDataType=sfix(16)  OutScaling=2^0
  MATLAB Fcn : MATLABFcn  MATLABFcn=u^2
  Mux1 : Mux  Inputs=3
  Mux2 : Mux  Inputs=3
  Mux3 : Mux  Inputs=3
  Product{,1..3} (4 alike) : Product  OutDataType=sfix(16)  OutScaling=2^0  RndMeth=Zero
  RMS1 : powerlib_extras/Measurements/RMS  DialogController=POWERSYS.PowerSysDialog  SystemSampleTime=-1  f1=50
  Scope1 : Scope  NumInputPorts=3
      settings: YMin=-1~-1~150000  YMax=1~1~320000
  Sine Wave : Sin  Amplitude=1  Bias=0  Frequency=100*pi  Phase=pi/2  Samples=10  SampleTime=0  Offset=0
  Sine Wave Function : Sin  Amplitude=1  Bias=0  Frequency=100*pi  Phase=0  Samples=10  SampleTime=0  Offset=0
  Sum : Sum  Inputs=|++  OutDataType=sfix(16)  OutScaling=2^0
  Sum1 : Sum  Inputs=|+++  OutDataType=sfix(16)  OutScaling=2^0
  Transport Delay : TransportDelay  DelayTime=.04/3
  Transport Delay2 : TransportDelay  DelayTime=.02/3
  Transport Delay3 : TransportDelay  DelayTime=.04/3
  Transport Delay4 : TransportDelay  DelayTime=.02/3
  eabc1+ : Outport  OutDataType=sfix(16)  OutScaling=2^0
  E+^2 : Outport  Port=2  OutDataType=sfix(16)  OutScaling=2^0
  wires:
  Transport Delay4/1 -> Sum1/3
  Transport Delay/1 -> Sum1/2
  Demux/1 -> Sum1/1
  Mux2/1 -> Gain1/1
  1st-Order  Filter5/1 -> Mux2/2
  1st-Order  Filter4/1 -> Mux2/1
  Product2/1 -> Demux2/1
  Demux2/3 -> 1st-Order  Filter1/1
  Demux2/2 -> 1st-Order  Filter5/1
  Demux2/1 -> 1st-Order  Filter4/1
  1st-Order  Filter1/1 -> Mux2/3
  Mux1/1 -> Gain/1
  1st-Order  Filter3/1 -> Mux1/2
  1st-Order  Filter2/1 -> Mux1/1
  Product/1 -> Demux1/1
  Demux1/3 -> 1st-Order  Filter/1
  Demux1/2 -> 1st-Order  Filter3/1
  Demux1/1 -> 1st-Order  Filter2/1
  Mux3/1 -> eabc1+/1
  Transport Delay3/1 -> Mux3/3
  Transport Delay2/1 -> Mux3/2
  Demux/3 -> Transport Delay4/1
  Sum1/1 -> Transport Delay2/1, RMS1/1, Mux3/1, Transport Delay3/1
  Demux/2 -> Transport Delay/1
  Sum/1 -> Demux/1
  Product3/1 -> Sum/2
  Product1/1 -> Sum/1
  Gain1/1 -> Product3/1
  Sine Wave/1 -> Product3/2, Product2/2
  Gain/1 -> Product1/1
  1st-Order  Filter/1 -> Mux1/3
  Sine Wave Function/1 -> Product1/2, Product/2
  In1/1 -> Product2/1, Product/1
  MATLAB Fcn/1 -> Scope1/3, E+^2/1
  RMS1/1 -> MATLAB Fcn/1

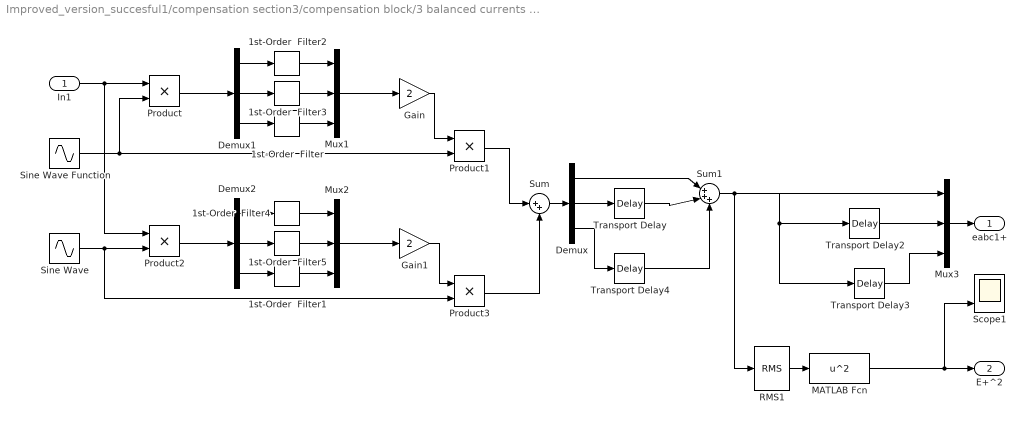
== system Improved_version_succesful1/compensation section3/compensation block/3 balanced currents /positive sequence1 ==
  In1 : Inport  OutDataType=sfix(16)  OutScaling=2^0
  1st-Order  Filter{,1,3,5} (4 alike) : powerlib_extras/Control  Blocks/1st-Order  Filter  DialogController=POWERSYS.PowerSysDialog  SystemSampleTime=-1  FilterType=Lowpass  Tc=.01  Initialize=off  Vac_Init=[0.8 -25 60]  Vdc_Init=-0.4  PlotResponse=off  param1=[1 500 1]
  1st-Order  Filter2 : powerlib_extras/Control  Blocks/1st-Order  Filter  DialogController=POWERSYS.PowerSysDialog  SystemSampleTime=-1  FilterType=Lowpass  Tc=.015  Initialize=off  Vac_Init=[0.8 -25 60]  Vdc_Init=-0.4  PlotResponse=off  param1=[1 500 1]
  1st-Order  Filter4 : powerlib_extras/Control  Blocks/1st-Order  Filter  DialogController=POWERSYS.PowerSysDialog  SystemSampleTime=-1  FilterType=Lowpass  Tc=.015  Initialize=off  Vac_Init=[0.8 -25 60]  Vdc_Init=-0.4  PlotResponse=off  param1=[1 500 1]
  Demux : Demux  Outputs=3
  Demux1 : Demux  Outputs=3
  Demux2 : Demux  Outputs=3
  Gain : Gain  Gain=2  ParameterDataType=sfix(16)  ParameterScaling=2^0  OutDataType=sfix(16)  OutScaling=2^0
  Gain1 : Gain  Gain=2  ParameterDataType=sfix(16)  ParameterScaling=2^0  OutDataType=sfix(16)  OutScaling=2^0
  MATLAB Fcn : MATLABFcn  MATLABFcn=u^2
  Mux1 : Mux  Inputs=3
  Mux2 : Mux  Inputs=3
  Mux3 : Mux  Inputs=3
  Product{,1..3} (4 alike) : Product  OutDataType=sfix(16)  OutScaling=2^0  RndMeth=Zero
  RMS1 : powerlib_extras/Measurements/RMS  DialogController=POWERSYS.PowerSysDialog  SystemSampleTime=-1  f1=50
  Scope1 : Scope  NumInputPorts=3
      settings: YMin=-1~-1~150000  YMax=1~1~320000
  Sine Wave : Sin  Amplitude=1  Bias=0  Frequency=100*pi  Phase=pi/2  Samples=10  SampleTime=0  Offset=0
  Sine Wave Function : Sin  Amplitude=1  Bias=0  Frequency=100*pi  Phase=0  Samples=10  SampleTime=0  Offset=0
  Sum : Sum  Inputs=|++  OutDataType=sfix(16)  OutScaling=2^0
  Sum1 : Sum  Inputs=|+++  OutDataType=sfix(16)  OutScaling=2^0
  Transport Delay : TransportDelay  DelayTime=.04/3
  Transport Delay2 : TransportDelay  DelayTime=.02/3
  Transport Delay3 : TransportDelay  DelayTime=.04/3
  Transport Delay4 : TransportDelay  DelayTime=.02/3
  eabc1+ : Outport  OutDataType=sfix(16)  OutScaling=2^0
  E+^2 : Outport  Port=2  OutDataType=sfix(16)  OutScaling=2^0
  wires:
  RMS1/1 -> MATLAB Fcn/1
  MATLAB Fcn/1 -> E+^2/1, Scope1/3
  In1/1 -> Product/1, Product2/1
  Sine Wave Function/1 -> Product/2, Product1/2
  1st-Order  Filter/1 -> Mux1/3
  Gain/1 -> Product1/1
  Sine Wave/1 -> Product2/2, Product3/2
  Gain1/1 -> Product3/1
  Product1/1 -> Sum/1
  Product3/1 -> Sum/2
  Sum/1 -> Demux/1
  Demux/2 -> Transport Delay/1
  Sum1/1 -> Transport Delay3/1, Mux3/1, RMS1/1, Transport Delay2/1
  Demux/3 -> Transport Delay4/1
  Transport Delay2/1 -> Mux3/2
  Transport Delay3/1 -> Mux3/3
  Mux3/1 -> eabc1+/1
  Demux1/1 -> 1st-Order  Filter2/1
  Demux1/2 -> 1st-Order  Filter3/1
  Demux1/3 -> 1st-Order  Filter/1
  Product/1 -> Demux1/1
  1st-Order  Filter2/1 -> Mux1/1
  1st-Order  Filter3/1 -> Mux1/2
  Mux1/1 -> Gain/1
  1st-Order  Filter1/1 -> Mux2/3
  Demux2/1 -> 1st-Order  Filter4/1
  Demux2/2 -> 1st-Order  Filter5/1
  Demux2/3 -> 1st-Order  Filter1/1
  Product2/1 -> Demux2/1
  1st-Order  Filter4/1 -> Mux2/1
  1st-Order  Filter5/1 -> Mux2/2
  Mux2/1 -> Gain1/1
  Demux/1 -> Sum1/1
  Transport Delay/1 -> Sum1/2
  Transport Delay4/1 -> Sum1/3

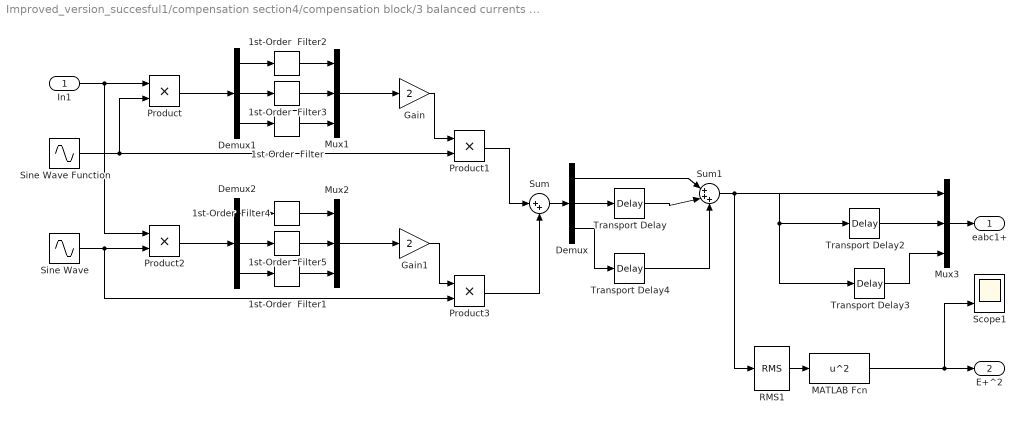
== system Improved_version_succesful1/compensation section4/compensation block/3 balanced currents /positive sequence1 ==
  In1 : Inport  OutDataType=sfix(16)  OutScaling=2^0
  1st-Order  Filter{,1,3,5} (4 alike) : powerlib_extras/Control  Blocks/1st-Order  Filter  DialogController=POWERSYS.PowerSysDialog  SystemSampleTime=-1  FilterType=Lowpass  Tc=.01  Initialize=off  Vac_Init=[0.8 -25 60]  Vdc_Init=-0.4  PlotResponse=off  param1=[1 500 1]
  1st-Order  Filter2 : powerlib_extras/Control  Blocks/1st-Order  Filter  DialogController=POWERSYS.PowerSysDialog  SystemSampleTime=-1  FilterType=Lowpass  Tc=.015  Initialize=off  Vac_Init=[0.8 -25 60]  Vdc_Init=-0.4  PlotResponse=off  param1=[1 500 1]
  1st-Order  Filter4 : powerlib_extras/Control  Blocks/1st-Order  Filter  DialogController=POWERSYS.PowerSysDialog  SystemSampleTime=-1  FilterType=Lowpass  Tc=.015  Initialize=off  Vac_Init=[0.8 -25 60]  Vdc_Init=-0.4  PlotResponse=off  param1=[1 500 1]
  Demux : Demux  Outputs=3
  Demux1 : Demux  Outputs=3
  Demux2 : Demux  Outputs=3
  Gain : Gain  Gain=2  ParameterDataType=sfix(16)  ParameterScaling=2^0  OutDataType=sfix(16)  OutScaling=2^0
  Gain1 : Gain  Gain=2  ParameterDataType=sfix(16)  ParameterScaling=2^0  OutDataType=sfix(16)  OutScaling=2^0
  MATLAB Fcn : MATLABFcn  MATLABFcn=u^2
  Mux1 : Mux  Inputs=3
  Mux2 : Mux  Inputs=3
  Mux3 : Mux  Inputs=3
  Product{,1..3} (4 alike) : Product  OutDataType=sfix(16)  OutScaling=2^0  RndMeth=Zero
  RMS1 : powerlib_extras/Measurements/RMS  DialogController=POWERSYS.PowerSysDialog  SystemSampleTime=-1  f1=50
  Scope1 : Scope  NumInputPorts=3
      settings: YMin=-1~-1~150000  YMax=1~1~320000
  Sine Wave : Sin  Amplitude=1  Bias=0  Frequency=100*pi  Phase=pi/2  Samples=10  SampleTime=0  Offset=0
  Sine Wave Function : Sin  Amplitude=1  Bias=0  Frequency=100*pi  Phase=0  Samples=10  SampleTime=0  Offset=0
  Sum : Sum  Inputs=|++  OutDataType=sfix(16)  OutScaling=2^0
  Sum1 : Sum  Inputs=|+++  OutDataType=sfix(16)  OutScaling=2^0
  Transport Delay : TransportDelay  DelayTime=.04/3
  Transport Delay2 : TransportDelay  DelayTime=.02/3
  Transport Delay3 : TransportDelay  DelayTime=.04/3
  Transport Delay4 : TransportDelay  DelayTime=.02/3
  eabc1+ : Outport  OutDataType=sfix(16)  OutScaling=2^0
  E+^2 : Outport  Port=2  OutDataType=sfix(16)  OutScaling=2^0
  wires:
  Transport Delay4/1 -> Sum1/3
  Transport Delay/1 -> Sum1/2
  Demux/1 -> Sum1/1
  Mux2/1 -> Gain1/1
  1st-Order  Filter5/1 -> Mux2/2
  1st-Order  Filter4/1 -> Mux2/1
  Product2/1 -> Demux2/1
  Demux2/3 -> 1st-Order  Filter1/1
  Demux2/2 -> 1st-Order  Filter5/1
  Demux2/1 -> 1st-Order  Filter4/1
  1st-Order  Filter1/1 -> Mux2/3
  Mux1/1 -> Gain/1
  1st-Order  Filter3/1 -> Mux1/2
  1st-Order  Filter2/1 -> Mux1/1
  Product/1 -> Demux1/1
  Demux1/3 -> 1st-Order  Filter/1
  Demux1/2 -> 1st-Order  Filter3/1
  Demux1/1 -> 1st-Order  Filter2/1
  Mux3/1 -> eabc1+/1
  Transport Delay3/1 -> Mux3/3
  Transport Delay2/1 -> Mux3/2
  Demux/3 -> Transport Delay4/1
  Sum1/1 -> Transport Delay2/1, RMS1/1, Mux3/1, Transport Delay3/1
  Demux/2 -> Transport Delay/1
  Sum/1 -> Demux/1
  Product3/1 -> Sum/2
  Product1/1 -> Sum/1
  Gain1/1 -> Product3/1
  Sine Wave/1 -> Product3/2, Product2/2
  Gain/1 -> Product1/1
  1st-Order  Filter/1 -> Mux1/3
  Sine Wave Function/1 -> Product1/2, Product/2
  In1/1 -> Product2/1, Product/1
  MATLAB Fcn/1 -> Scope1/3, E+^2/1
  RMS1/1 -> MATLAB Fcn/1
